simulink model "deltasigma_code_gen"  (R2017b)
settings: Solver=FixedStepAuto  StartTime=0.0  StopTime=10e-3  FixedStep=T  RelTol=1e-3
InitFcn:
  | T=1/50e6;
  | tau = 0.01e-3;
libraries: simulink x1
settings Model: Creator=roman  LastModifiedBy=roman

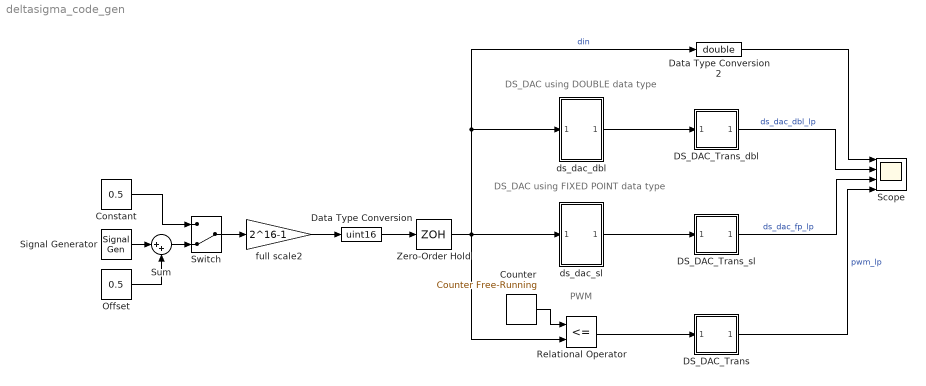
== system deltasigma_code_gen ==
  note: DS_DAC using DOUBLE data type
  note: DS_DAC using FIXED POINT data type
  note: PWM
  Constant : Constant  Value=0.5
  Counter : simulink/Sources/Counter Free-Running  NumBits=16  tsamp=T
  DS_DAC_Trans : Subsystem
  DS_DAC_Trans_dbl : Subsystem
  DS_DAC_Trans_sl : Subsystem
  Data Type Conversion : DataTypeConversion  OutDataTypeStr=uint16
  Data Type Conversion2 : DataTypeConversion  OutDataTypeStr=double
  Offset : Constant  Value=0.5
  Relational Operator : RelationalOperator  Operator=<=  OutDataTypeStr=boolean  RndMeth=Simplest
  Scope : Scope  NumInputPorts=4
  Signal Generator : SignalGenerator  Amplitude=0.5  Frequency=100
  Sum : Sum  Inputs=|++
  Switch : ManualSwitch  CurrentSetting=0
  Zero-Order Hold : ZeroOrderHold  SampleTime=T
  ds_dac_dbl : Subsystem
  ds_dac_sl : Subsystem
  full scale2 : Gain  Gain=2^16-1
  wires:
  Sum/1 -> Switch/2
  Switch/1 -> full scale2/1
  Signal Generator/1 -> Sum/1
  Offset/1 -> Sum/2
  Constant/1 -> Switch/1
  full scale2/1 -> Data Type Conversion/1
  Data Type Conversion/1 -> Zero-Order Hold/1
  Counter/1 -> Relational Operator/1
  Zero-Order Hold/1 -> Data Type Conversion2/1, ds_dac_dbl/1(din), Relational Operator/2, ds_dac_sl/1(din)  "din"
  Data Type Conversion2/1 -> Scope/1
  Relational Operator/1 -> DS_DAC_Trans/1(In1)
  DS_DAC_Trans/1(Out1) -> Scope/4  "pwm_lp"
  DS_DAC_Trans_sl/1(Out1) -> Scope/3  "ds_dac_fp_lp"
  DS_DAC_Trans_dbl/1(Out1) -> Scope/2  "ds_dac_dbl_lp"
  ds_dac_dbl/1(dout) -> DS_DAC_Trans_dbl/1(In1)
  ds_dac_sl/1(dout) -> DS_DAC_Trans_sl/1(In1)

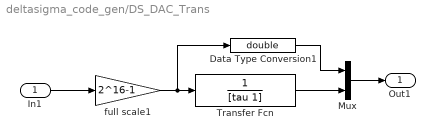
== system deltasigma_code_gen/DS_DAC_Trans ==
  In1 : Inport
  Data Type Conversion1 : DataTypeConversion  OutDataTypeStr=double
  Mux : Mux  Inputs=2
  Transfer Fcn : TransferFcn  Denominator=[tau 1]
  full scale1 : Gain  Gain=2^16-1  OutDataTypeStr=double
  Out1 : Outport
  wires:
  full scale1/1 -> Transfer Fcn/1, Data Type Conversion1/1
  Transfer Fcn/1 -> Mux/2
  Mux/1 -> Out1/1
  Data Type Conversion1/1 -> Mux/1
  In1/1 -> full scale1/1

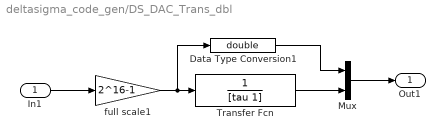
== system deltasigma_code_gen/DS_DAC_Trans_dbl ==
  In1 : Inport
  Data Type Conversion1 : DataTypeConversion  OutDataTypeStr=double
  Mux : Mux  Inputs=2
  Transfer Fcn : TransferFcn  Denominator=[tau 1]
  full scale1 : Gain  Gain=2^16-1  OutDataTypeStr=double
  Out1 : Outport
  wires:
  full scale1/1 -> Transfer Fcn/1, Data Type Conversion1/1
  Transfer Fcn/1 -> Mux/2
  Mux/1 -> Out1/1
  Data Type Conversion1/1 -> Mux/1
  In1/1 -> full scale1/1

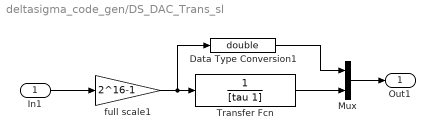
== system deltasigma_code_gen/DS_DAC_Trans_sl ==
  In1 : Inport
  Data Type Conversion1 : DataTypeConversion  OutDataTypeStr=double
  Mux : Mux  Inputs=2
  Transfer Fcn : TransferFcn  Denominator=[tau 1]
  full scale1 : Gain  Gain=2^16-1  OutDataTypeStr=double
  Out1 : Outport
  wires:
  full scale1/1 -> Transfer Fcn/1, Data Type Conversion1/1
  Transfer Fcn/1 -> Mux/2
  Mux/1 -> Out1/1
  Data Type Conversion1/1 -> Mux/1
  In1/1 -> full scale1/1

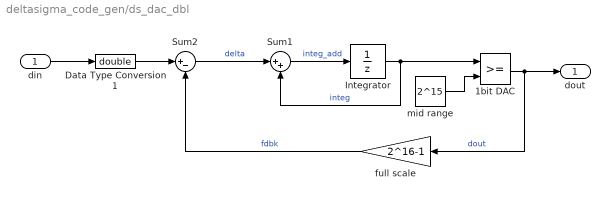
== system deltasigma_code_gen/ds_dac_dbl ==
  din : Inport
  1bit DAC : RelationalOperator  OutDataTypeStr=boolean  RndMeth=Simplest
  Data Type Conversion1 : DataTypeConversion  OutDataTypeStr=double
  Integrator : UnitDelay  SampleTime=T
  Sum1 : Sum  Inputs=|++
  Sum2 : Sum  Inputs=|+-
  full scale : Gain  Gain=2^16-1  OutDataTypeStr=double
  mid range : Constant  Value=2^15  OutDataTypeStr=double  SampleTime=T
  dout : Outport
  wires:
  Integrator/1 -> Sum1/2, 1bit DAC/1  "integ"
  full scale/1 -> Sum2/2  "fdbk"
  Sum2/1 -> Sum1/1  "delta"
  Sum1/1 -> Integrator/1  "integ_add"
  mid range/1 -> 1bit DAC/2
  din/1 -> Data Type Conversion1/1
  1bit DAC/1 -> dout/1, full scale/1  "dout"
  Data Type Conversion1/1 -> Sum2/1

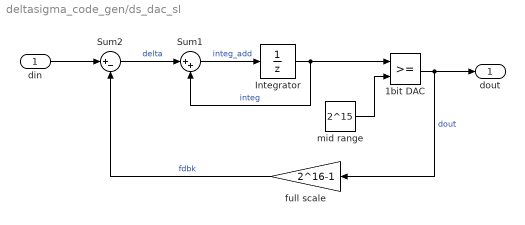
== system deltasigma_code_gen/ds_dac_sl ==
  din : Inport
  1bit DAC : RelationalOperator  OutDataTypeStr=boolean  RndMeth=Simplest
  Integrator : UnitDelay  SampleTime=T
  Sum1 : Sum  Inputs=|++  OutDataTypeStr=fixdt(1,18,0)
  Sum2 : Sum  Inputs=|+-  OutDataTypeStr=fixdt(1,17,0)
  full scale : Gain  Gain=2^16-1  OutDataTypeStr=uint16
  mid range : Constant  Value=2^15  OutDataTypeStr=fixdt(1,18,0)  SampleTime=T
  dout : Outport
  wires:
  Integrator/1 -> Sum1/2, 1bit DAC/1  "integ"
  full scale/1 -> Sum2/2  "fdbk"
  Sum2/1 -> Sum1/1  "delta"
  Sum1/1 -> Integrator/1  "integ_add"
  mid range/1 -> 1bit DAC/2
  1bit DAC/1 -> dout/1, full scale/1  "dout"
  din/1 -> Sum2/1
